simulink model "SRM1"  (R2021b)
settings: Solver=ode23t  StartTime=0.0  StopTime=10.0  MaxStep=1e-5  RelTol=1e-3
settings Model: Creator=Len_comp  LastModifiedBy=Len_comp
settings SolverCC: ZeroCrossControl=DisableAll

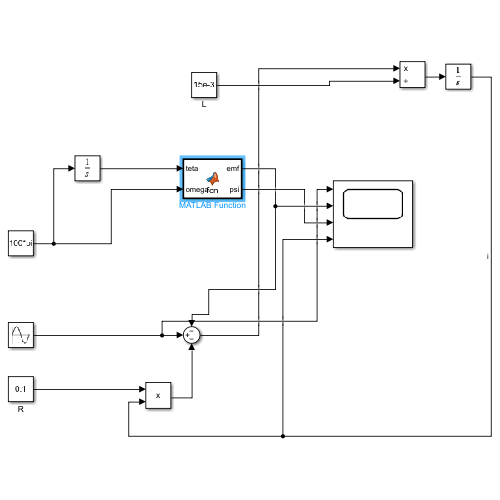
[thumbnail: Simulink's stored preview of the top-level diagram]
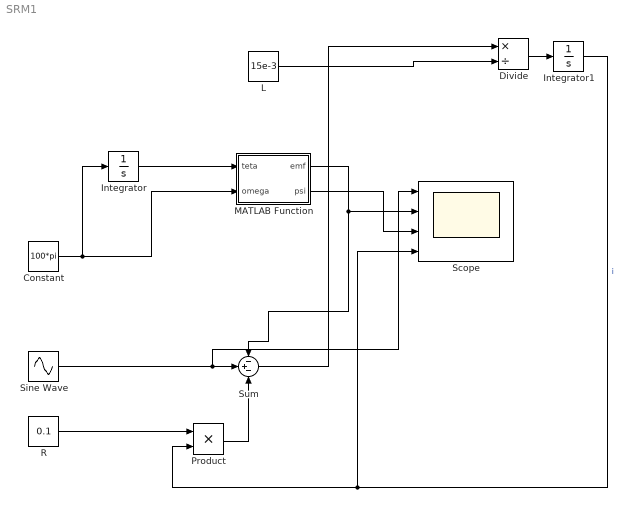
== system SRM1 ==
  Constant : Constant  Value=100*pi
  Divide : Product  Inputs=*/
  Integrator : Integrator
  Integrator1 : Integrator
  L : Constant  Value=15e-3
  MATLAB Function : MATLAB Function  TreatAsAtomicUnit=on
  Product : Product
  R : Constant  Value=0.1
  Scope : Scope  NumInputPorts=4
  Sine Wave : Sin  Amplitude=50  Frequency=100*pi  SampleTime=0
  Sum : Sum  Inputs=-+-
  wires:
  Constant/1 -> Integrator/1, MATLAB Function/2(omega)
  Integrator/1 -> MATLAB Function/1(teta)
  MATLAB Function/1(emf) -> Sum/1, Scope/2
  MATLAB Function/2(psi) -> Scope/3
  Sine Wave/1 -> Scope/1, Sum/2
  Product/1 -> Sum/3
  Integrator1/1 -> Scope/4, Product/2  "i"
  R/1 -> Product/1
  Sum/1 -> Divide/1
  Divide/1 -> Integrator1/1
  L/1 -> Divide/2

== matlab function SRM1/MATLAB Function ==
  data: teta input; emf output; omega input; psi output
function [emf, psi] = fcn(teta, omega)
%harmonic representation of EMF and flux in the machine

psi1 = 0.15;
psi3 = 0.0;

emf = omega * psi1 * sin(teta) + omega * 3 * psi3 * sin(3 * teta);
psi = psi1 * cos(teta) + psi3 * cos(3 * teta);
